simulink model "STM32_G4_ESC_blinky"  (R2023a)
settings: Solver=FixedStepAuto  StartTime=0.0  StopTime=10.0  RelTol=1e-3  EnableMultiTasking=on
undefined symbols (not defined in the file): append
libraries: stm32f4xxblockslib x2, simulink x1, stm32blockslib x1
settings Model: Creator=n10201378  LastModifiedBy=n10201378
settings SolverCC: AutoInsertRateTranBlk=on
settings OptimizationCC: EnhancedBackFolding=on  PassReuseOutputArgsAs=Individual arguments  ZeroExternalMemoryAtStartup=off  ZeroInternalMemoryAtStartup=off  MaxStackSize=64  OptimizeBlockOrder=speed  DifferentSizesBufferReuse=on  OptimizationCustomize=off  EfficientTunableParamExpr=on
settings DebuggingCC: ParameterTunabilityLossMsg=error
settings HardwareCC: ProdBitPerPointer=32  ProdBitPerSizeT=32  ProdBitPerPtrDiffT=32  ProdLargestAtomicInteger=Long  ProdLargestAtomicFloat=Double  ProdWordSize=32  ProdLongLongMode=on  ProdHWDeviceType=ARM Compatible->ARM Cortex
settings SFSimCC: MATLABDynamicMemAlloc=off
settings RTWCC: Description=Embedded Coder  SystemTargetFile=ert.tlc  HardwareBoard=STM32G4xx Based  TemplateMakefile=ert_default_tmf  Toolchain=GNU Tools for ARM Embedded Processors
settings CodeAppCC: ForceParamTrailComments=on  IgnoreCustomStorageClasses=off  OperatorAnnotations=on  SimulinkDataObjDesc=on  SFDataObjDesc=on  InsertBlockDesc=on
settings ERTTargetCC: CodeReplacementLibrary=ARM Cortex-M  ExtModeTransport=3  ExtModeStaticAlloc=on  ExtModeStaticAllocSize=2048  ExtModeMexFile=ext_xcp  ExtModeIntrfLevel=Level2 - Open

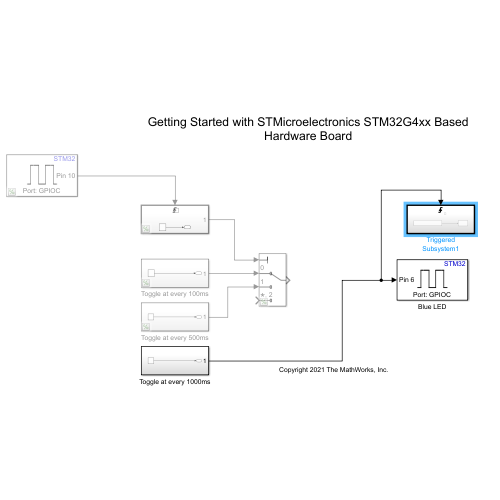
[thumbnail: Simulink's stored preview of the top-level diagram]
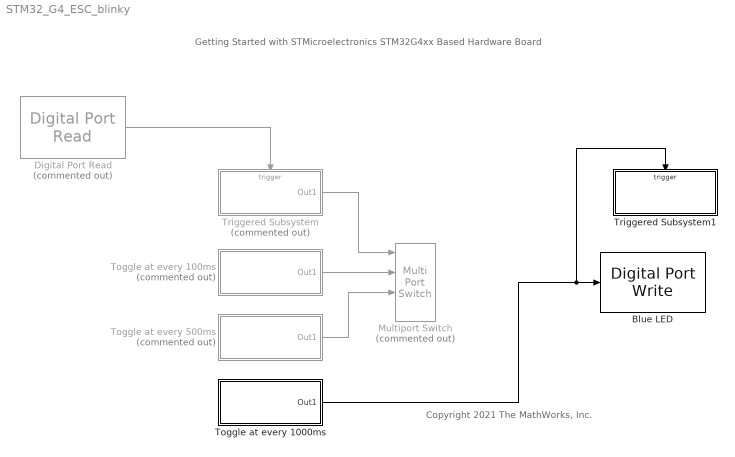
== system STM32_G4_ESC_blinky ==
  note: Getting Started with STMicroelectronics STM32G4xx Based Hardware Board
  note: Copyright 2021 The MathWorks, Inc.
  Blue LED : stm32f4xxblockslib/Digital Port Write  PortName=GPIOC  PinNumber=6  ReadOperation=off  IOAsArray=off  EnableSimPort=off
  Digital Port Read : stm32f4xxblockslib/Digital Port Read  Commented=on  PortName=GPIOC  PinNumber=10  ReadOperation=on  IOAsArray=off  SampleTime=-1  EnableSimPort=off
      settings: LibrarySourceBlock=stm32g4xxblockslib/Digital Port Read
  Multiport Switch : MultiPortSwitch  Commented=on  DataPortOrder=Zero-based contiguous  zeroidx=on  SaturateOnIntegerOverflow=off  InputSameDT=off
  Toggle at every 1000ms : Subsystem
  Toggle at every 100ms : Subsystem  Commented=on
  Toggle at every 500ms : Subsystem  Commented=on
  Triggered Subsystem : Subsystem  Commented=on  TreatAsAtomicUnit=on
  Triggered Subsystem1 : Subsystem  TreatAsAtomicUnit=on
  wires:
  Toggle at every 500ms/1(Out1) -> Multiport Switch/3
  Digital Port Read/1 -> Triggered Subsystem/Trigger
  Toggle at every 100ms/1(Out1) -> Multiport Switch/2
  Triggered Subsystem/1(Out1) -> Multiport Switch/1
  Toggle at every 1000ms/1(Out1) -> Triggered Subsystem1/Trigger, Blue LED/1

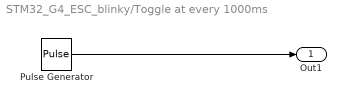
== system STM32_G4_ESC_blinky/Toggle at every 1000ms ==
  Pulse Generator : DiscretePulseGenerator
  Out1 : Outport
  wires:
  Pulse Generator/1 -> Out1/1

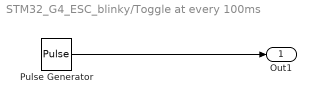
== system STM32_G4_ESC_blinky/Toggle at every 100ms ==
  Pulse Generator : DiscretePulseGenerator  SampleTime=0.1
  Out1 : Outport
  wires:
  Pulse Generator/1 -> Out1/1

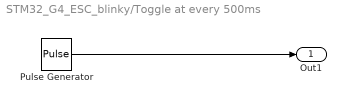
== system STM32_G4_ESC_blinky/Toggle at every 500ms ==
  Pulse Generator : DiscretePulseGenerator  SampleTime=0.5
  Out1 : Outport
  wires:
  Pulse Generator/1 -> Out1/1

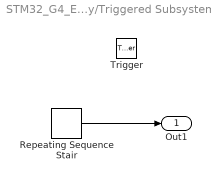
== system STM32_G4_ESC_blinky/Triggered Subsystem ==
  Trigger : TriggerPort  VariantControl=(inherit)
  Repeating Sequence Stair : simulink/Sources/Repeating Sequence Stair  OutValues=[1 2 0]  tsamp=-1  OutMin=[]  OutMax=[]  OutDataTypeStr=double  OutputDataTypeScalingMode=double  OutDataType=fixdt(0,8)  ConRadixGroup=Best Precision: Vector-wise  OutScaling=2^-12
  Out1 : Outport
  wires:
  Repeating Sequence Stair/1 -> Out1/1

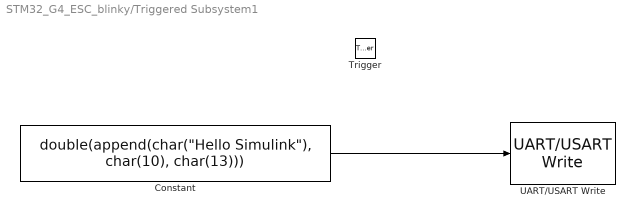
== system STM32_G4_ESC_blinky/Triggered Subsystem1 ==
  Trigger : TriggerPort  VariantControl=(inherit)
  Constant : Constant  Value="double(append(char(\"Hello Simulink\"), char(10), char(13)))"  OutDataTypeStr=uint8
  UART/USART Write : stm32blockslib/UART//USART Write  Priority=1  UARTModule=USART2  LengthOfDataToSend=off  BlockingMode=off  BlockingTimeout=0.1  OutputStatus=off
      settings: LibrarySourceBlock=stm32g4xxblockslib/UART//USART Write
  wires:
  Constant/1 -> UART/USART Write/1
